simulink model "adrc_quandruple_tanks"  (Simulink 6.0)
settings: Solver=ode45  StartTime=0.0  StopTime=10.0  RelTol=1e-3
undefined symbols (not defined in the file or in its folder): A1, a1, A2, a2, A3, a3, A4, a4, g, gama1, gama2, h10, h20, h30, h40, k1, k2
settings Model: LastModifiedBy=dell

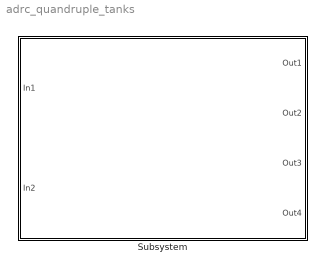
== system adrc_quandruple_tanks ==
  Subsystem : Subsystem

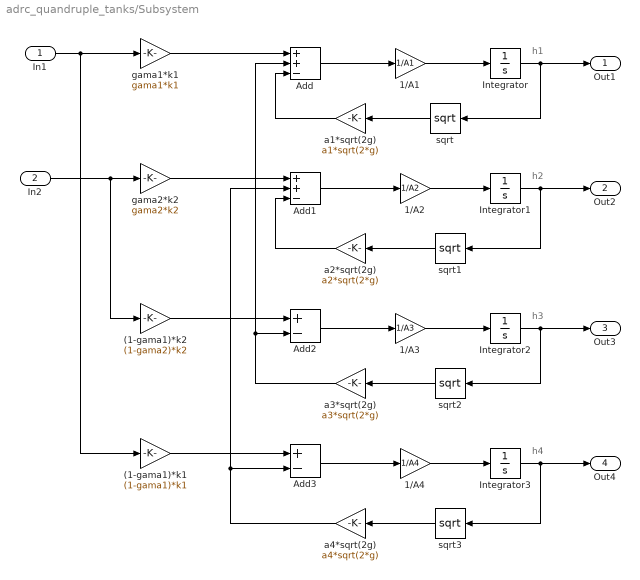
== system adrc_quandruple_tanks/Subsystem ==
  note: h1
  note: h2
  note: h3
  note: h4
  In1 : Inport  Port=1  OutDataType=fixdt(1,16,0)  OutScaling=[]  LatchInput=off
  In2 : Inport  Port=2  OutDataType=fixdt(1,16,0)  OutScaling=[]  LatchInput=off
  (1-gama1)*k1 : Gain  Gain=(1-gama1)*k1
  (1-gama1)*k2 : Gain  Gain=(1-gama2)*k2
  1/A1 : Gain  Gain=1/A1
  1/A2 : Gain  Gain=1/A2
  1/A3 : Gain  Gain=1/A3
  1/A4 : Gain  Gain=1/A4
  Add : Sum  Inputs=++-  OutScaling=2^-10
  Add1 : Sum  Inputs=++-  OutScaling=2^-10
  Add2 : Sum  Inputs=+-  OutScaling=2^-10
  Add3 : Sum  Inputs=+-  OutScaling=2^-10
  Integrator : Integrator  InitialCondition=h10
  Integrator1 : Integrator  InitialCondition=h20
  Integrator2 : Integrator  InitialCondition=h30
  Integrator3 : Integrator  InitialCondition=h40
  a1*sqrt(2g) : Gain  Orientation=left  Gain=a1*sqrt(2*g)
  a2*sqrt(2g) : Gain  Orientation=left  Gain=a2*sqrt(2*g)
  a3*sqrt(2g) : Gain  Orientation=left  Gain=a3*sqrt(2*g)
  a4*sqrt(2g) : Gain  Orientation=left  Gain=a4*sqrt(2*g)
  gama1*k1 : Gain  Gain=gama1*k1
  gama2*k2 : Gain  Gain=gama2*k2
  sqrt{,1..3} (4 alike) : Math  Orientation=left  Operator=sqrt  SaturateOnIntegerOverflow=on
  Out1 : Outport  OutDataType=fixdt(1,16,0)  OutScaling=[]
  Out2 : Outport  Port=2  OutDataType=fixdt(1,16,0)  OutScaling=[]
  Out3 : Outport  Port=3  OutDataType=fixdt(1,16,0)  OutScaling=[]
  Out4 : Outport  Port=4  OutDataType=fixdt(1,16,0)  OutScaling=[]
  wires:
  Integrator/1 -> Out1/1, sqrt/1
  sqrt/1 -> a1*sqrt(2g)/1
  Integrator1/1 -> Out2/1, sqrt1/1
  sqrt1/1 -> a2*sqrt(2g)/1
  Integrator2/1 -> Out3/1, sqrt2/1
  sqrt2/1 -> a3*sqrt(2g)/1
  Integrator3/1 -> Out4/1, sqrt3/1
  sqrt3/1 -> a4*sqrt(2g)/1
  1/A1/1 -> Integrator/1
  1/A2/1 -> Integrator1/1
  1/A3/1 -> Integrator2/1
  1/A4/1 -> Integrator3/1
  Add/1 -> 1/A1/1
  gama1*k1/1 -> Add/1
  a1*sqrt(2g)/1 -> Add/3
  Add1/1 -> 1/A2/1
  Add2/1 -> 1/A3/1
  Add3/1 -> 1/A4/1
  a3*sqrt(2g)/1 -> Add2/2, Add/2
  a2*sqrt(2g)/1 -> Add1/3
  gama2*k2/1 -> Add1/1
  (1-gama1)*k1/1 -> Add3/1
  (1-gama1)*k2/1 -> Add2/1
  a4*sqrt(2g)/1 -> Add1/2, Add3/2
  In2/1 -> gama2*k2/1, (1-gama1)*k2/1
  In1/1 -> gama1*k1/1, (1-gama1)*k1/1
